simulink model "unitdelay_vect_test"  (Simulink 7.2)
settings: Solver=ode45  StartTime=0.0  StopTime=10.0  RelTol=1e-3
settings Model: Creator=arnaud  LastModifiedBy=arnaud
settings DataIOCC: SaveFormat=Structure

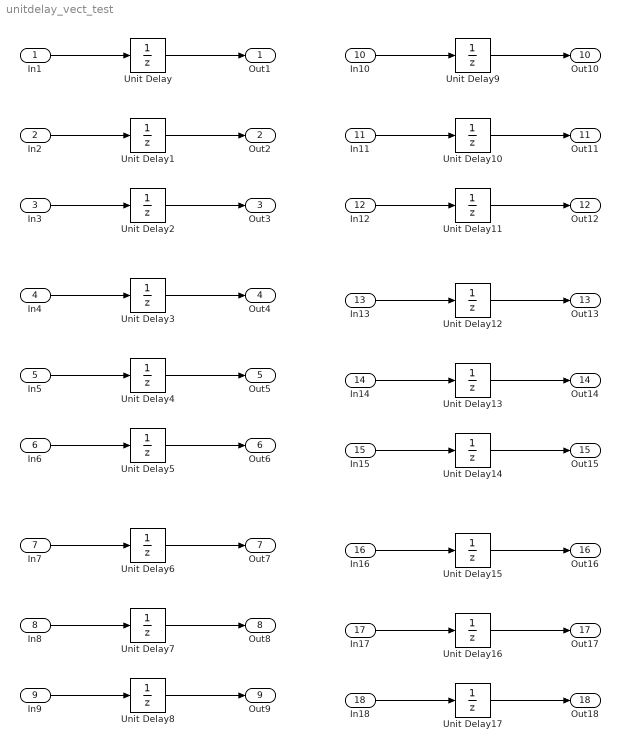
== system unitdelay_vect_test ==
  In1 : Inport  PortDimensions=2  DataType=double  OutDataType=sfix(16)  OutScaling=2^0  OutDataTypeStr=double
  In2 : Inport  Port=2  PortDimensions=2  DataType=double  OutDataType=sfix(16)  OutScaling=2^0  OutDataTypeStr=double
  In3 : Inport  Port=3  PortDimensions=2  OutDataType=sfix(16)  OutScaling=2^0
  In4 : Inport  Port=4  PortDimensions=2  DataType=int8  OutDataType=sfix(16)  OutScaling=2^0  OutDataTypeStr=int8
  In5 : Inport  Port=5  PortDimensions=2  DataType=int8  OutDataType=sfix(16)  OutScaling=2^0  OutDataTypeStr=int8
  In6 : Inport  Port=6  PortDimensions=2  DataType=int8  OutDataType=sfix(16)  OutScaling=2^0  OutDataTypeStr=int8
  In7 : Inport  Port=7  PortDimensions=2  DataType=boolean  OutDataType=sfix(16)  OutScaling=2^0  OutDataTypeStr=boolean
  In8 : Inport  Port=8  PortDimensions=2  DataType=boolean  OutDataType=sfix(16)  OutScaling=2^0  OutDataTypeStr=boolean
  In9 : Inport  Port=9  PortDimensions=2  DataType=boolean  OutDataType=sfix(16)  OutScaling=2^0  OutDataTypeStr=boolean
  In10 : Inport  Port=10  PortDimensions=2  DataType=double  OutDataType=sfix(16)  OutScaling=2^0  OutDataTypeStr=double
  In11 : Inport  Port=11  PortDimensions=2  DataType=double  OutDataType=sfix(16)  OutScaling=2^0  OutDataTypeStr=double
  In12 : Inport  Port=12  PortDimensions=2  OutDataType=sfix(16)  OutScaling=2^0
  In13 : Inport  Port=13  PortDimensions=2  DataType=int8  OutDataType=sfix(16)  OutScaling=2^0  OutDataTypeStr=int8
  In14 : Inport  Port=14  PortDimensions=2  DataType=int8  OutDataType=sfix(16)  OutScaling=2^0  OutDataTypeStr=int8
  In15 : Inport  Port=15  PortDimensions=2  DataType=int8  OutDataType=sfix(16)  OutScaling=2^0  OutDataTypeStr=int8
  In16 : Inport  Port=16  PortDimensions=2  DataType=boolean  OutDataType=sfix(16)  OutScaling=2^0  OutDataTypeStr=boolean
  In17 : Inport  Port=17  PortDimensions=2  DataType=boolean  OutDataType=sfix(16)  OutScaling=2^0  OutDataTypeStr=boolean
  In18 : Inport  Port=18  PortDimensions=2  DataType=boolean  OutDataType=sfix(16)  OutScaling=2^0  OutDataTypeStr=boolean
  Unit Delay : UnitDelay
  Unit Delay1 : UnitDelay  X0=0.0
  Unit Delay{9..10,12..13,15..16} (6 alike) : UnitDelay  X0=[0 2]
  Unit Delay11 : UnitDelay  X0=[true false]
  Unit Delay14 : UnitDelay  X0=[false true]
  Unit Delay17 : UnitDelay  X0=[false true]
  Unit Delay2 : UnitDelay  X0=true
  Unit Delay3 : UnitDelay
  Unit Delay4 : UnitDelay  X0=0.0
  Unit Delay5 : UnitDelay  X0=true
  Unit Delay6 : UnitDelay
  Unit Delay7 : UnitDelay  X0=0.0
  Unit Delay8 : UnitDelay  X0=true
  Out1 : Outport  OutDataType=sfix(16)  OutScaling=2^0
  Out2 : Outport  Port=2  OutDataType=sfix(16)  OutScaling=2^0
  Out3 : Outport  Port=3  OutDataType=sfix(16)  OutScaling=2^0
  Out4 : Outport  Port=4  OutDataType=sfix(16)  OutScaling=2^0
  Out5 : Outport  Port=5  OutDataType=sfix(16)  OutScaling=2^0
  Out6 : Outport  Port=6  OutDataType=sfix(16)  OutScaling=2^0
  Out7 : Outport  Port=7  OutDataType=sfix(16)  OutScaling=2^0
  Out8 : Outport  Port=8  OutDataType=sfix(16)  OutScaling=2^0
  Out9 : Outport  Port=9  OutDataType=sfix(16)  OutScaling=2^0
  Out10 : Outport  Port=10  OutDataType=sfix(16)  OutScaling=2^0
  Out11 : Outport  Port=11  OutDataType=sfix(16)  OutScaling=2^0
  Out12 : Outport  Port=12  OutDataType=sfix(16)  OutScaling=2^0
  Out13 : Outport  Port=13  OutDataType=sfix(16)  OutScaling=2^0
  Out14 : Outport  Port=14  OutDataType=sfix(16)  OutScaling=2^0
  Out15 : Outport  Port=15  OutDataType=sfix(16)  OutScaling=2^0
  Out16 : Outport  Port=16  OutDataType=sfix(16)  OutScaling=2^0
  Out17 : Outport  Port=17  OutDataType=sfix(16)  OutScaling=2^0
  Out18 : Outport  Port=18  OutDataType=sfix(16)  OutScaling=2^0
  wires:
  In1/1 -> Unit Delay/1
  Unit Delay/1 -> Out1/1
  In2/1 -> Unit Delay1/1
  Unit Delay1/1 -> Out2/1
  In3/1 -> Unit Delay2/1
  Unit Delay2/1 -> Out3/1
  In4/1 -> Unit Delay3/1
  Unit Delay3/1 -> Out4/1
  In5/1 -> Unit Delay4/1
  Unit Delay4/1 -> Out5/1
  In6/1 -> Unit Delay5/1
  Unit Delay5/1 -> Out6/1
  In7/1 -> Unit Delay6/1
  Unit Delay6/1 -> Out7/1
  In8/1 -> Unit Delay7/1
  Unit Delay7/1 -> Out8/1
  In9/1 -> Unit Delay8/1
  Unit Delay8/1 -> Out9/1
  In10/1 -> Unit Delay9/1
  Unit Delay9/1 -> Out10/1
  In11/1 -> Unit Delay10/1
  Unit Delay10/1 -> Out11/1
  In12/1 -> Unit Delay11/1
  Unit Delay11/1 -> Out12/1
  In13/1 -> Unit Delay12/1
  Unit Delay12/1 -> Out13/1
  In14/1 -> Unit Delay13/1
  Unit Delay13/1 -> Out14/1
  In15/1 -> Unit Delay14/1
  Unit Delay14/1 -> Out15/1
  In16/1 -> Unit Delay15/1
  Unit Delay15/1 -> Out16/1
  In17/1 -> Unit Delay16/1
  Unit Delay16/1 -> Out17/1
  In18/1 -> Unit Delay17/1
  Unit Delay17/1 -> Out18/1
